simulink model "power_FlybackConverter_hardware"  (R2018a)
settings: Solver=VariableStepAuto  StartTime=0.0  StopTime=0.004  MaxStep=1e-8  RelTol=1e-4  EnableMultiTasking=on
libraries: powerlib x17
Description:
  | Copyright 2008-2018 The MathWorks, Inc.
settings Model: Creator=MathWorks  LastModifiedBy=FAHRİ TÜREDİ
settings SolverCC: SolverResetMethod=Robust
settings DataIOCC: ReturnWorkspaceOutputs=on
settings OptimizationCC: LifeSpan=inf
settings DebuggingCC: ReadBeforeWriteMsg=DisableAll  WriteAfterWriteMsg=DisableAll  WriteAfterReadMsg=DisableAll  MultiTaskDSMMsg=none  SFUnexpectedBacktrackingDiag=warning  SFNoUnconditionalDefaultTransitionDiag=warning  SFExecutionAtInitializationDiag=none
settings ModelReferenceCC: UpdateModelReferenceTargets=IfOutOfDate
settings SFSimCC: SFSimEcho=off
settings CodeAppCC: StateflowObjectComments=on
settings GRTTargetCC: TargetLangStandard=C89/C90 (ANSI)  GeneratePreprocessorConditionals=Disable all
settings ConfigComp: CovMetricSettings=dw  CovHtmlReporting=on  CovSaveCumulativeToWorkspaceVar=on  CovSaveSingleToWorkspaceVar=on  CovExternalEMLEnable=off
settings SimscapeCC: SimscapeNormalizeSystem=off  SimscapeNominalValues={1, 'bar'; 1, 'cm^3/s'; 1, 'bar*kg/s'; 1, 'kJ/kg'; 1, 'kW'; }

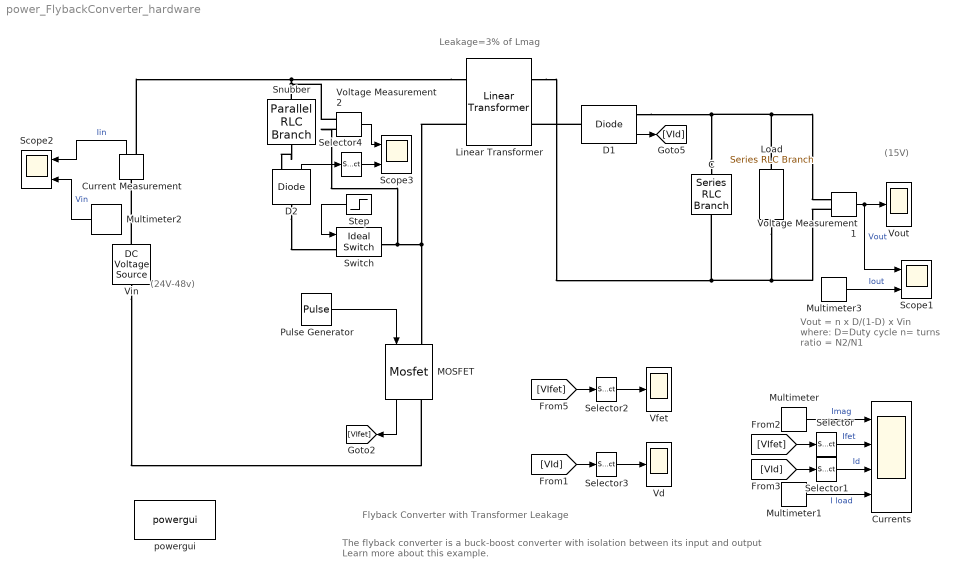
== system power_FlybackConverter_hardware ==
  note: (15V)
  note: Leakage=3% of Lmag
  note: Vout = n x D/(1-D) x Vin
      | where: D=Duty cycle
      | n= turns ratio = N2/N1
  note: (24V-48v)
  note: Flyback Converter with Transformer Leakage
  note: The flyback converter is a buck-boost converter with isolation between its input and output
      |
      | Learn more about this example.
  C : powerlib/Elements/Series RLC Branch  LConnTagsString=__new0  RConnTagsString=__new0  BranchType=RC  Resistance=20e-3  Inductance=200e-6  SetiL0=off  InitialCurrent=0  Capacitance=200e-6  Setx0=off  InitialVoltage=0  Measurements=None
  Current Measurement : powerlib/Measurements/Current Measurement  PhasorSimulation=off  OutputType=Complex  PSBequivalent=0
  Currents : Scope  NumInputPorts=4
  D1 : powerlib/Power Electronics/Diode  Ron=0.001  Lon=0  Vf=0.7  IC=0  UseSnubber=off  Rs=500  Cs=250e-9  Measurements=on
  D2 : powerlib/Power Electronics/Diode  Ron=1e-3  Lon=0  Vf=0  IC=0  UseSnubber=off  Rs=inf  Cs=0  Measurements=on
  Linear Transformer : powerlib/Elements/Linear Transformer  UNITS=SI  NominalPower=[ 100 45000 ]  winding1=[200 26.753e-3 0.8601e-6]  winding2=[105.263 14.223e-3 0]  ThreeWindings=off  winding3=[3.15e+05 3.969e+07 6316.9]  RmLm=[1e4 28.67e-6]  Measurements=Magnetization current  DataType=on
  Load : powerlib/Elements/Series RLC Branch  LConnTagsString=__new0  RConnTagsString=__new0  BranchType=R  Resistance=15/4  Inductance=200e-6  SetiL0=off  InitialCurrent=0  Capacitance=400e-6  Setx0=off  InitialVoltage=0  Measurements=Branch current
  MOSFET : powerlib/Power Electronics/Mosfet  Ron=0.1  Lon=0  Rd=0.01  Vfd=0  IC=0  Rs=1e6  Cs=inf  Measurements=on
  Multimeter : powerlib/Measurements/Multimeter  PhasorSimulation=off  OutputType=Complex  sel=4  L=5  Gain=1  yselected={'Imag: Linear Transformer'};  PSBOutputType=1  PSBequivalent=0  AxesSetting=[0,0.1,-100,100]  Display=0  SavedBlockNames=-11
  Multimeter1 : powerlib/Measurements/Multimeter  PhasorSimulation=off  OutputType=Complex  sel=2  L=5  Gain=1  yselected={'Ib: Load'};  PSBOutputType=1  PSBequivalent=0  AxesSetting=[0,0.1,-100,100]  Display=0  SavedBlockNames=-11
  Multimeter2 : powerlib/Measurements/Multimeter  PhasorSimulation=off  OutputType=Complex  sel=1  L=5  Gain=1  yselected={'Usrc: Vin'};  PSBOutputType=1  PSBequivalent=0  AxesSetting=[0,0.1,-100,100]  Display=0  SavedBlockNames=-11
  Multimeter3 : powerlib/Measurements/Multimeter  PhasorSimulation=off  OutputType=Complex  sel=2  L=5  Gain=1  yselected={'Ib: Load'};  PSBOutputType=1  PSBequivalent=0  AxesSetting=[0,0.1,-100,100]  Display=0  SavedBlockNames=-11
  Pulse Generator : DiscretePulseGenerator  PulseType=Time based  Period=1/45000  PulseWidth=57
  Scope1 : Scope  NumInputPorts=2
  Scope2 : Scope  NumInputPorts=2
  Scope3 : Scope  NumInputPorts=2
  Selector : Selector  InputPortWidth=2  IndexOptions=Index vector (dialog)  Indices=1  OutputSizes=1
  Selector1 : Selector  InputPortWidth=2  IndexOptions=Index vector (dialog)  Indices=1  OutputSizes=1
  Selector2 : Selector  InputPortWidth=2  IndexOptions=Index vector (dialog)  Indices=2  OutputSizes=1
  Selector3 : Selector  InputPortWidth=2  IndexOptions=Index vector (dialog)  Indices=2  OutputSizes=1
  Selector4 : Selector  InputPortWidth=2  IndexOptions=Index vector (dialog)  Indices=1  OutputSizes=1
  Snubber : powerlib/Elements/Parallel RLC Branch  LConnTagsString=a  RConnTagsString=__new0  BranchType=RC  Resistance=10e3  Inductance=1e-3  SetiL0=off  InitialCurrent=0  Capacitance=47e-9  Setx0=off  InitialVoltage=0  Measurements=None
  Step : Step  Time=0  SampleTime=0
  Switch : powerlib/Power Electronics/Ideal Switch  Ron=0.001  Lon=0  IC=0  Rs=inf  Cs=0  Measurements=off
  Vd : Scope
  Vfet : Scope
  Vin : powerlib/Electrical Sources/DC Voltage Source  Amplitude=24  Measurements=Voltage
  Voltage Measurement1 : powerlib/Measurements/Voltage Measurement  PhasorSimulation=off  OutputType=Complex  PSBequivalent=0
  Voltage Measurement2 : powerlib/Measurements/Voltage Measurement  PhasorSimulation=off  OutputType=Complex  PSBequivalent=0
  Vout : Scope
  powergui : powerlib/powergui  Priority=1  SimulationMode=Continuous  SampleTime=50e-6  frequency=60  Iterations=50  frequencyindice=0  Pbase=100e6  ErrMax=1e-4  UnitsV=kV  UnitsW=MW  buscounter=0  FunctionMessages=off  echomessages=off  EnableUseOfTLC=off  CurrentSourceSwitches=off  DisableSnubberDevices=off  DisableRonSwitches=off  DisableVfSwitches=off  DisplayEquations=off  SolverType=Tustin/Backward Euler (TBE)  Interpol=off  ExternalGateDelay=off  methode=off  Ts=100  x0status=blocks  SPID=on  SwTol=0  HookPort=off  RestoreLinks=warning  ResistiveCurrentMeasurement=off  Frange=[0:2:500]  Ylog=off  Xlog=on  ShowGrid=off  save=off  variable=ZData  structure=0  ZoomFFT=off  StartTime=0.0  cycles=1  DisplayStyle=1  fundamental=60  FreqAxis=off  MaxFrequency=1000  frequencyindicesteady=1  RmsSteady=1  display=off
  wires:
  Pulse Generator/1 -> MOSFET/1
  Voltage Measurement1/1 -> Vout/1, Scope1/1  "Vout"
  MOSFET/1 -> [VIfet]
  D1/1 -> [VId]
  Multimeter/1 -> Currents/1  "Imag"
  Selector/1 -> Currents/2  "Ifet"
  [VIfet] -> Selector/1
  Selector1/1 -> Currents/3  "Id"
  [VId] -> Selector1/1
  Multimeter1/1 -> Currents/4  "I load"
  Selector2/1 -> Vfet/1
  [VIfet] -> Selector2/1
  Step/1 -> Switch/1
  [VId] -> Selector3/1
  Selector3/1 -> Vd/1
  Multimeter2/1 -> Scope2/2  "Vin"
  Current Measurement/1 -> Scope2/1  "Iin"
  Multimeter3/1 -> Scope1/2  "Iout"
  Voltage Measurement2/1 -> Scope3/1
  Selector4/1 -> Scope3/2
  D2/1 -> Selector4/1
  connections:
  C/LConn1 -- Voltage Measurement1/LConn1 -- Load/LConn1 -- D1/RConn1
  Load/RConn1 -- Voltage Measurement1/LConn2 -- Linear Transformer/RConn1 -- C/RConn1
  Linear Transformer/LConn2 -- Voltage Measurement2/LConn2 -- Switch/RConn1 -- MOSFET/LConn1
  D1/LConn1 -- Linear Transformer/RConn2
  Snubber/RConn1 -- D2/RConn1
  Vin/LConn1 -- MOSFET/RConn1
  Linear Transformer/LConn1 -- Voltage Measurement2/LConn1 -- Snubber/LConn1 -- Current Measurement/RConn1
  D2/LConn1 -- Switch/LConn1
  Vin/RConn1 -- Current Measurement/LConn1
